simulink model "project_model_part2_detector2"  (R2020a)
settings: Solver=VariableStepAuto  StartTime=0.0  StopTime=350  RelTol=1e-3
undefined symbols (not defined in the file or in its folder): Discrete, Time
libraries: ctrlSharedLib x1
settings Model: Creator=Admin  LastModifiedBy=Shreya
settings DataIOCC: ReturnWorkspaceOutputs=off
settings DebuggingCC: ArithmeticOperatorsInVariantConditions=warning
settings SFSimCC: SimUseLocalCustomCode=off  CustomCodeUndefinedFunction=UseInterfaceOnly
settings RTWCC: RTWUseLocalCustomCode=off

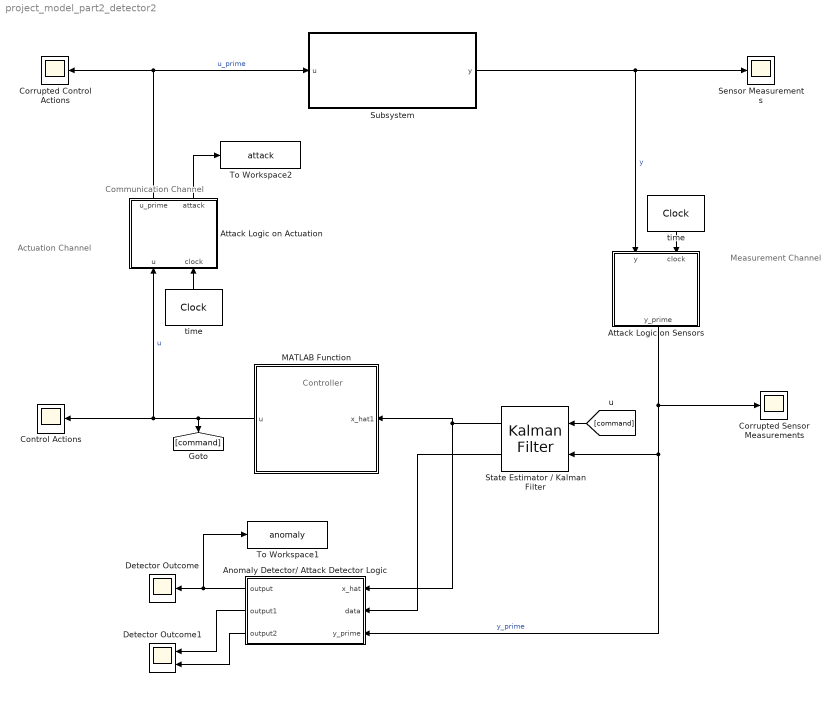
== system project_model_part2_detector2 ==
  note: Controller
  note: Communication Channel
  note: Measurement Channel
  note: Actuation Channel
  Anomaly Detector/ Attack Detector Logic : MATLAB Function  TreatAsAtomicUnit=on
  Attack Logic on Actuation : MATLAB Function  TreatAsAtomicUnit=on
  Attack Logic on Sensors : MATLAB Function  TreatAsAtomicUnit=on
  Control Actions : Scope
  Corrupted Control Actions : Scope
  Corrupted Sensor Measurements : Scope
  Detector Outcome : Scope
  Detector Outcome1 : Scope  NumInputPorts=2
  MATLAB Function : MATLAB Function  TreatAsAtomicUnit=on
  "Sensor Measurements " : Scope
  State Estimator / Kalman Filter : ctrlSharedLib/Kalman Filter  TimeDomain=Discrete-Time  UseCurrentEstimator=on  ModelSource=Individual A, B, C, D matrices  ModelSourceVariable=sys  A="[1.0000    0.0001   -0.0010;0.5747    1.0000   -0.0003;0.0162    0.0000    1.0000]"  B="[0.1   -0.2; -0.0536    0.0332;0.1955   -0.5294];"  C=[1 0 0;0 1 0]  D=[0 0;0 0]  NumberOfStates=2  NumberOfInputs=2  NumberOfOutputs=2  InitialEstimateSource=Dialog  X0=[0;0;0]  P0=10  UseK=off  UseGH=off  NumberOfProcessNoiseInputs=2  G=1  TimeInvariantG=on  H=0  TimeInvariantH=on  Q=0.00001*eye(3)  TimeInvariantQ=on  R=0.00008*eye(2)  TimeInvariantR=on  N=0  TimeInvariantN=on  AddInputPort=on  AddEnablePort=off  OutputEstimatedY=off  OutputP=on  Ts=-1
  Subsystem : Subsystem
  To Workspace1 : ToWorkspace  VariableName=anomaly  SaveFormat=Timeseries  SampleTime=0.1
      settings: Save2DSignal=2-D array (concatenate along first dimension)
  To Workspace2 : ToWorkspace  VariableName=attack  SaveFormat=Timeseries  SampleTime=0.1
      settings: Save2DSignal=2-D array (concatenate along first dimension)
  time : DigitalClock  SampleTime=0.1
  "time " : DigitalClock  SampleTime=0.1
  wires:
  Anomaly Detector/ Attack Detector Logic/1(output) -> To Workspace1/1, Detector Outcome/1
  "time "/1 -> Attack Logic on Sensors/2(clock)
  Attack Logic on Sensors/1(y_prime) -> Anomaly Detector/ Attack Detector Logic/3(y_prime), State Estimator / Kalman Filter/2, Corrupted Sensor Measurements/1  "y_prime"
  MATLAB Function/1(u) -> Attack Logic on Actuation/1(u), Control Actions/1, [command]  "u"
  time/1 -> Attack Logic on Actuation/2(clock)
  Attack Logic on Actuation/1(u_prime) -> Subsystem/1(u), Corrupted Control Actions/1  "u_prime"
  [command] -> State Estimator / Kalman Filter/1
  Subsystem/1(y) -> Attack Logic on Sensors/1(y), "Sensor Measurements "/1  "y"
  State Estimator / Kalman Filter/1 -> Anomaly Detector/ Attack Detector Logic/1(x_hat), MATLAB Function/1(x_hat1)
  State Estimator / Kalman Filter/2 -> Anomaly Detector/ Attack Detector Logic/2(data)
  Anomaly Detector/ Attack Detector Logic/2(output1) -> Detector Outcome1/1
  Anomaly Detector/ Attack Detector Logic/3(output2) -> Detector Outcome1/2
  Attack Logic on Actuation/2(attack) -> To Workspace2/1

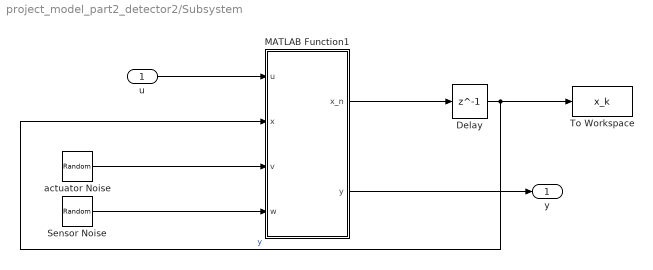
== system project_model_part2_detector2/Subsystem ==
  u : Inport
  Delay : Delay  DelayLength=1  InitialCondition=[0 0.1 0.2]
  MATLAB Function1 : MATLAB Function  TreatAsAtomicUnit=on
  Sensor Noise : RandomNumber  Mean=[0 0]  Variance=[0.00008 0.00008]  Seed=[randi(100) randi(100)]
  To Workspace : ToWorkspace  VariableName=x_k  SaveFormat=Timeseries  SampleTime=-1
  actuator Noise : RandomNumber  Mean=[0 0 0]  Variance=[0.00001 0.00001 0.00001]  Seed=[randi(100) randi(100) randi(100)]
  y : Outport  VectorParamsAs1DForOutWhenUnconnected=off
  wires:
  u/1 -> MATLAB Function1/1(u)
  MATLAB Function1/1(x_n) -> Delay/1
  MATLAB Function1/2(y) -> y/1
  Sensor Noise/1 -> MATLAB Function1/4(w)
  actuator Noise/1 -> MATLAB Function1/3(v)
  Delay/1 -> To Workspace/1, MATLAB Function1/2(x)  "y"

== matlab function project_model_part2_detector2/Attack Logic on Sensors ==
  data: y input; y_prime output; clock input
function y_prime = fcn(y,clock)
% this function should contain the attacker action on the sensor
% measurements
y_prime = y;
end

== matlab function project_model_part2_detector2/MATLAB Function ==
  data: x_hat1 input; u output
function u  = Controller(x_hat1)
%two tanks model 
    

%controller gain
K =[17.1291   -1.1789   -6.5335; -0.1248   -2.9385   -2.5082];
u=-K*(x_hat1);

== matlab function project_model_part2_detector2/Attack Logic on Actuation ==
  data: u input; u_prime output; clock input; attack output
function [u_prime,attack] = fcn(u,clock)
% this function should contain the attacker action on the control inputs
%Attack logic on Actuation channel
%here u_a is attack vector
if clock >= 0 && clock < 40
    u_a = transpose([0 ,0]);
    attack = 0;
elseif clock >= 40 && clock < 50
    u_a = transpose([-0.18 ,-0.18]);
    attack = 1;
elseif clock >= 50 && clock < 300
    u_a = transpose([0 ,0]);
    attack = 0;
elseif clock >= 300 && clock < 310
    u_a = transpose([-0.21 ,-0.21]);
    attack = 1;
else
    u_a = transpose([0 ,0]);
    attack = 0;
end
u_prime = u + u_a;
end

== matlab function project_model_part2_detector2/Anomaly Detector// Attack Detector Logic ==
  data: x_hat input; output output; data input; output1 output; output2 output; y_prime input
function [output,output1,output2] = Detector(x_hat,data,y_prime)
% this function should contain the detection strategy

%CUSUM (Cumulative Sum) is a sequential analysis technique which is used 
%to aggregate the error over an adaptive window to protech the system
%against samll, but persistent attacks.
C = [1 0 0; 0 1 0];
R = 0.00008*eye(2);
%Here P is error covarience.
P = data;
sigma = (C * P * (transpose(C))) + R;
r = y_prime - (C * x_hat);
% Choosen Distance Measure but it is possible to drive CUSUM with any other distance measure
z = transpose(r) * (inv(sigma) * r);
%Here b is 'bias parameter'. For the tightest detection b is similar to P(state estimater error Covarience)
%Since z >= 0, the bias parameter b prevents the inherent growth due to the sum of nonnegative number.
%bias b must be selected properly based on the properties of the distance measure.
b = 2;
persistent s;
if isempty(s)
    %intially Cumulative sum is zero
    s = 0;
end
%Here beta is threshold value. 
%Once the bias is chosen, the threshold bita must be selected to fulfill a required false alarm rate.
beta = 13.5;
if s <= beta
    s = max([0,s + z - b]);
    output = 0;
else
    s = 0;
    output = 1;
end
output1 = s;
output2 = beta;
end

== matlab function project_model_part2_detector2/Subsystem/MATLAB Function1 ==
  data: x_n output; u input; y output; x input; v input; w input
function [x_n, y] = fcn(u, x, v, w)

A=[1.0000    0.0001   -0.0010;0.5747    1.0000   -0.0003;0.0162    0.0000    1.0000];
B = [0.1   -0.2; -0.0536    0.0332;0.1955   -0.5294];

C=[1 0 0;0 1 0];
D=[0 0;0 0];


x_n = A*x + B*u + v;
y = C*x + D*u + w;
